simulink model "Single_Phase_PWM_Dual_Inverter_grid_R2023a"  (R2023a)
settings: Solver=ode45  StartTime=0.0  StopTime=0.2  RelTol=1e-3
libraries: spsMosfetLib x8, spsSeriesRLCBranchLib x7, spsCurrentMeasurementLib x3, spsDCVoltageSourceLib x2, spsPLLLib x2, spsPWMGenerator2LevelLib x2, spsVoltageMeasurementLib x2, spsACVoltageSourceLib x1, spspowerguiLib x1
settings Model: Creator=JD  LastModifiedBy=JD
settings DebuggingCC: UnconnectedInputMsg=warning  UnconnectedOutputMsg=warning  UnconnectedLineMsg=warning
settings ModelReferenceCC: EnableRefExpFcnMdlSchedulingChecks=on
settings RTWCC: DLArmComputeVersion=19.05

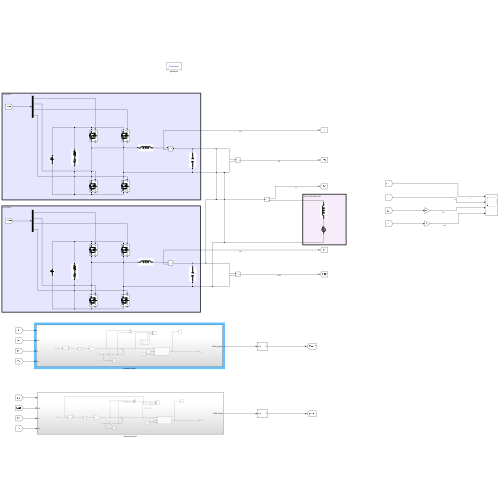
[thumbnail: Simulink's stored preview of the top-level diagram]
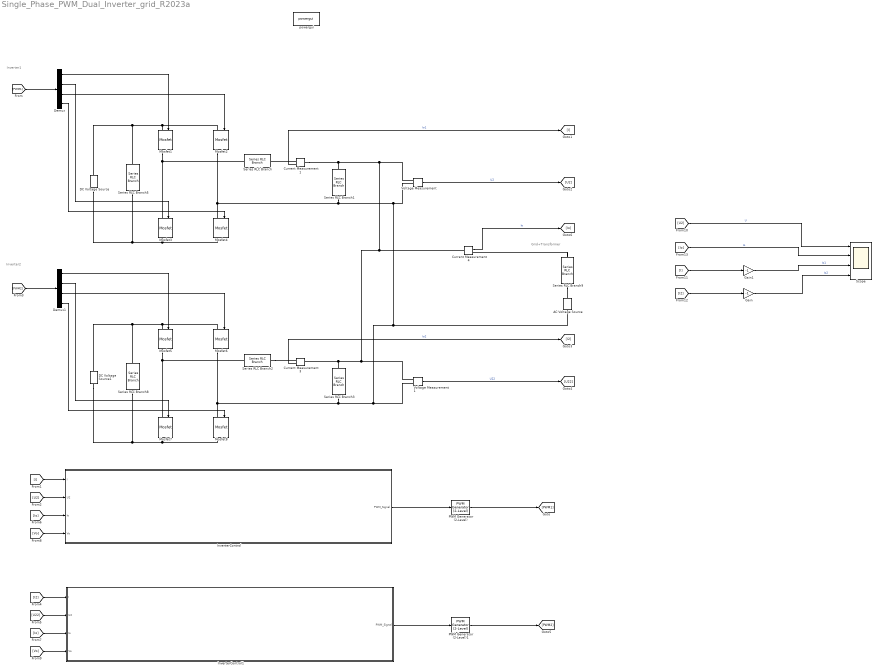
== system Single_Phase_PWM_Dual_Inverter_grid_R2023a ==
  note: Grid+Transformer
  note: Inverter2
  note: Inverter1
  AC Voltage Source : spsACVoltageSourceLib/AC Voltage Source  Amplitude=24*sqrt(2)  Phase=0  Frequency=50  SampleTime=0  Measurements=None  BusType=swing  Pref=10e3  Qref=0  Qmin=-inf  Qmax=+inf
  Current Measurement1 : spsCurrentMeasurementLib/Current Measurement  PhasorSimulation=off  OutputType=Complex  PSBequivalent=0
  Current Measurement3 : spsCurrentMeasurementLib/Current Measurement  PhasorSimulation=off  OutputType=Complex  PSBequivalent=0
  Current Measurement4 : spsCurrentMeasurementLib/Current Measurement  PhasorSimulation=off  OutputType=Complex  PSBequivalent=0
  DC Voltage Source : spsDCVoltageSourceLib/DC Voltage Source  Amplitude=48  Measurements=None
  DC Voltage Source1 : spsDCVoltageSourceLib/DC Voltage Source  Amplitude=48  Measurements=None
  Demux : Demux
  Demux1 : Demux
  Gain : Gain  Gain=-1
  Gain1 : Gain  Gain=-1
  InverterControl : Subsystem
  InverterControl1 : Subsystem
  Mosfet{1..8} (8 alike) : spsMosfetLib/Mosfet  Ron=0.1  Lon=0  Rd=0.01  Vfd=0  IC=0  Rs=1e5  Cs=inf  Measurements=on
  PWM Generator (2-Level) : spsPWMGenerator2LevelLib/PWM Generator (2-Level)  ModulatorType=Single-phase full-bridge (4 pulses)  ModulatorMode=Unsynchronized  Fc=20000  Pc=90  nF=27  MinMax="[ -1  1 ]"  SamplingTechnique=Natural  ModulatingSignals=off  m=0.8  Freq=60  Phase=0  Ts=0  ShowCarrierOutport=off
  PWM Generator (2-Level)1 : spsPWMGenerator2LevelLib/PWM Generator (2-Level)  ModulatorType=Single-phase full-bridge (4 pulses)  ModulatorMode=Unsynchronized  Fc=20000  Pc=90  nF=27  MinMax="[ -1  1 ]"  SamplingTechnique=Natural  ModulatingSignals=off  m=0.8  Freq=60  Phase=0  Ts=0  ShowCarrierOutport=off
  Scope : Scope  NumInputPorts=4
  Series RLC Branch : spsSeriesRLCBranchLib/Series RLC Branch  LConnTagsString=__new0  RConnTagsString=__new0  BranchType=L  Resistance=1  Inductance=1e-3  SetiL0=off  InitialCurrent=0  Capacitance=1e-6  Setx0=off  InitialVoltage=0  Measurements=None
  Series RLC Branch1 : spsSeriesRLCBranchLib/Series RLC Branch  LConnTagsString=__new0  RConnTagsString=__new0  BranchType=C  Resistance=1  Inductance=1e-3  SetiL0=off  InitialCurrent=0  Capacitance=4.7e-6  Setx0=off  InitialVoltage=0  Measurements=None
  Series RLC Branch2 : spsSeriesRLCBranchLib/Series RLC Branch  LConnTagsString=__new0  RConnTagsString=__new0  BranchType=L  Resistance=1  Inductance=1e-3  SetiL0=off  InitialCurrent=0  Capacitance=1e-6  Setx0=off  InitialVoltage=0  Measurements=None
  Series RLC Branch3 : spsSeriesRLCBranchLib/Series RLC Branch  LConnTagsString=__new0  RConnTagsString=__new0  BranchType=C  Resistance=1  Inductance=1e-3  SetiL0=off  InitialCurrent=0  Capacitance=4.7e-6  Setx0=off  InitialVoltage=0  Measurements=None
  Series RLC Branch5 : spsSeriesRLCBranchLib/Series RLC Branch  LConnTagsString=__new0  RConnTagsString=__new0  BranchType=RC  Resistance=0.0001  Inductance=1e-3  SetiL0=off  InitialCurrent=0  Capacitance=940e-6  Setx0=off  InitialVoltage=0  Measurements=None
  Series RLC Branch8 : spsSeriesRLCBranchLib/Series RLC Branch  LConnTagsString=__new0  RConnTagsString=__new0  BranchType=RC  Resistance=0.0001  Inductance=1e-3  SetiL0=off  InitialCurrent=0  Capacitance=940e-6  Setx0=off  InitialVoltage=0  Measurements=None
  Series RLC Branch9 : spsSeriesRLCBranchLib/Series RLC Branch  LConnTagsString=__new0  RConnTagsString=__new0  BranchType=L  Resistance=1  Inductance=100e-6  SetiL0=off  InitialCurrent=0  Capacitance=1e-6  Setx0=off  InitialVoltage=0  Measurements=None
  Voltage Measurement : spsVoltageMeasurementLib/Voltage Measurement  PhasorSimulation=off  OutputType=Complex  PSBequivalent=0
  Voltage Measurement1 : spsVoltageMeasurementLib/Voltage Measurement  PhasorSimulation=off  OutputType=Complex  PSBequivalent=0
  powergui : spspowerguiLib/powergui  Priority=1  SimulationMode=Continuous  SampleTime=1e-6  frequency=60  Iterations=50  frequencyindice=0  Pbase=100e6  ErrMax=1e-4  UnitsV=kV  UnitsW=MW  buscounter=0  FunctionMessages=off  echomessages=off  EnableUseOfTLC=off  CurrentSourceSwitches=off  DisableSnubberDevices=off  DisableRonSwitches=off  DisableVfSwitches=off  DisplayEquations=off  AutomaticDiscreteSolvers=off  SolverType=Tustin/Backward Euler (TBE)  Interpol=off  ExternalGateDelay=off  methode=off  Ts=100  x0status=blocks  SPID=on  SwTol=0  HookPort=off  NonlinearTolerance=1e-4  nMaxIteration=100  ContinueOnMaxIteration=off  RestoreLinks=warning  ResistiveCurrentMeasurement=off  Frange=[0:2:500]  Ylog=off  Xlog=on  ShowGrid=off  save=off  variable=ZData  structure=0  ZoomFFT=off  StartTime=0.0  cycles=1  DisplayStyle=1  fundamental=60  FreqAxis=off  MaxFrequency=1000  frequencyindicesteady=1  RmsSteady=1  display=off
  wires:
  Voltage Measurement/1 -> [U2]  "U2"
  [PWM1] -> Demux/1
  Demux/1 -> Mosfet1/1
  Demux/2 -> Mosfet3/1
  Demux/3 -> Mosfet2/1
  Demux/4 -> Mosfet4/1
  PWM Generator (2-Level)/1 -> [PWM1]
  Current Measurement1/1 -> [I]  "Io1"
  [I] -> InverterControl/1(I)
  [U2] -> InverterControl/2(U2)
  InverterControl/1(PWM_Signal) -> PWM Generator (2-Level)/1
  Current Measurement3/1 -> [I2]  "Io2"
  Demux1/4 -> Mosfet8/1
  Demux1/3 -> Mosfet6/1
  Demux1/2 -> Mosfet7/1
  Demux1/1 -> Mosfet5/1
  [PWM2] -> Demux1/1
  Voltage Measurement1/1 -> [U22]  "U22"
  InverterControl1/1(PWM_Signal) -> PWM Generator (2-Level)1/1
  [U22] -> InverterControl1/2(U2)
  [I2] -> InverterControl1/1(I)
  Current Measurement4/1 -> [Io]  "Io"
  [Io] -> InverterControl/3(Io)
  [Io] -> InverterControl1/3(Io)
  [Vo] -> InverterControl/4(Vo)
  [Vo] -> InverterControl1/4(Vo)
  PWM Generator (2-Level)1/1 -> [PWM2]
  [U2] -> Scope/1  "U"
  [I] -> Gain1/1
  [I2] -> Gain/1
  [Io] -> Scope/2  "Io"
  Gain1/1 -> Scope/3  "Io1"
  Gain/1 -> Scope/4  "Io2"
  connections:
  Mosfet2/LConn1 -- DC Voltage Source/RConn1 -- Series RLC Branch5/LConn1 -- Mosfet1/LConn1
  Mosfet4/RConn1 -- DC Voltage Source/LConn1 -- Series RLC Branch5/RConn1 -- Mosfet3/RConn1
  Mosfet1/RConn1 -- Mosfet3/LConn1 -- Series RLC Branch/LConn1
  Current Measurement1/RConn1 -- Series RLC Branch/RConn1
  Mosfet6/RConn1 -- Mosfet8/LConn1 -- Series RLC Branch3/RConn1 -- AC Voltage Source/LConn1 -- Mosfet2/RConn1 -- Mosfet4/LConn1 -- Series RLC Branch1/RConn1 -- Voltage Measurement/LConn2 -- Voltage Measurement1/LConn2
  Series RLC Branch9/LConn1 -- Current Measurement4/RConn1
  Mosfet6/LConn1 -- DC Voltage Source1/RConn1 -- Series RLC Branch8/LConn1 -- Mosfet5/LConn1
  Mosfet8/RConn1 -- Series RLC Branch8/RConn1 -- DC Voltage Source1/LConn1 -- Mosfet7/RConn1
  Mosfet5/RConn1 -- Series RLC Branch2/LConn1 -- Mosfet7/LConn1
  Series RLC Branch2/RConn1 -- Current Measurement3/RConn1
  Voltage Measurement1/LConn1 -- Current Measurement4/LConn1 -- Current Measurement1/LConn1 -- Series RLC Branch1/LConn1 -- Voltage Measurement/LConn1 -- Current Measurement3/LConn1 -- Series RLC Branch3/LConn1
  Series RLC Branch9/RConn1 -- AC Voltage Source/RConn1

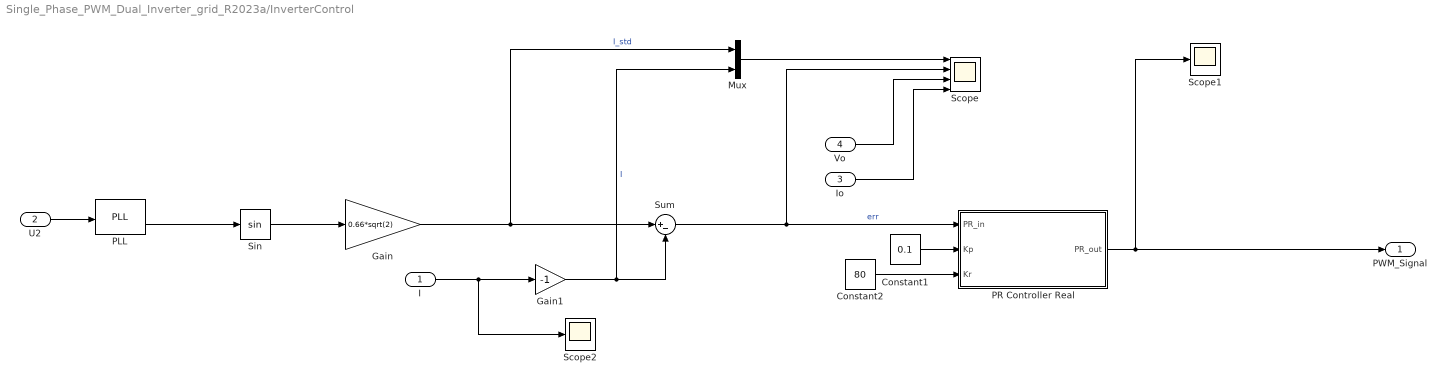
== system Single_Phase_PWM_Dual_Inverter_grid_R2023a/InverterControl ==
  I : Inport
  U2 : Inport  Port=2
  Io : Inport  Port=3
  Vo : Inport  Port=4
  Constant1 : Constant  Value=0.1
  Constant2 : Constant  Value=80
  Gain : Gain  Gain=0.66*sqrt(2)
  Gain1 : Gain  Gain=-1
  Mux : Mux  Inputs=2
  PLL : spsPLLLib/PLL  Fmin=45  Par_Init=[0, 50]  ParK=[180, 3200, 1]  TcD=1e-4  MaxRateChangeFreq=12  FilterCutOffFreq=25  Ts=0  AGC=on
  PR Controller Real : Subsystem
  Scope : Scope  NumInputPorts=4
  Scope1 : Scope
  Scope2 : Scope
  Sin : Trigonometry
  Sum : Sum  Inputs=|+-
  PWM_Signal : Outport
  wires:
  Constant1/1 -> PR Controller Real/2(Kp)
  Constant2/1 -> PR Controller Real/3(Kr)
  Mux/1 -> Scope/1
  Sum/1 -> PR Controller Real/1(PR_in), Scope/2  "err"
  PR Controller Real/1(PR_out) -> PWM_Signal/1, Scope1/1
  I/1 -> Scope2/1, Gain1/1
  Io/1 -> Scope/4
  Gain1/1 -> Sum/2, Mux/2  "I"
  U2/1 -> PLL/1
  PLL/2 -> Sin/1
  Sin/1 -> Gain/1
  Gain/1 -> Mux/1, Sum/1  "I_std"
  Vo/1 -> Scope/3

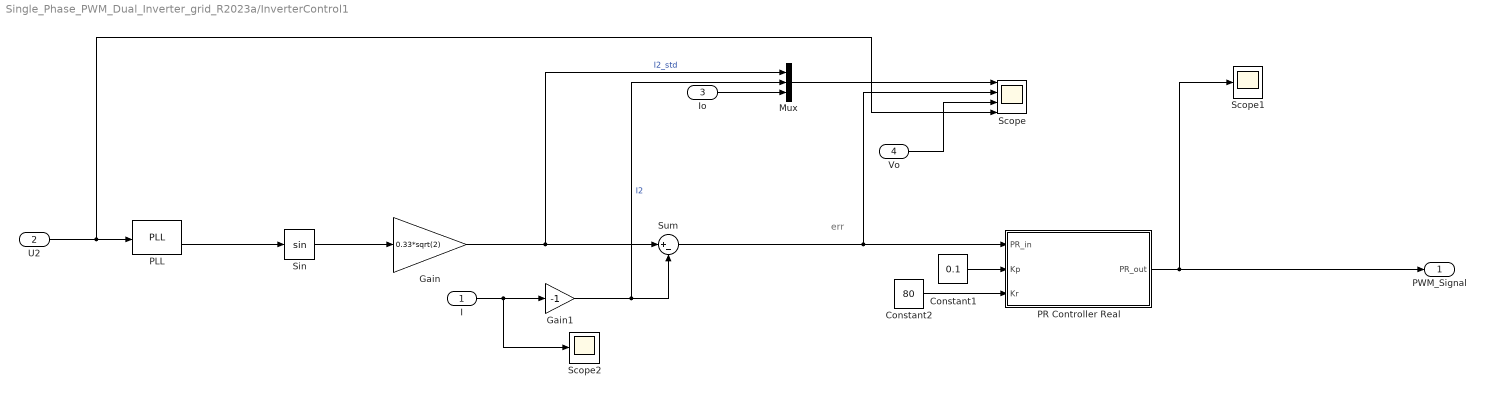
== system Single_Phase_PWM_Dual_Inverter_grid_R2023a/InverterControl1 ==
  note: err
  I : Inport
  U2 : Inport  Port=2
  Io : Inport  Port=3
  Vo : Inport  Port=4
  Constant1 : Constant  Value=0.1
  Constant2 : Constant  Value=80
  Gain : Gain  Gain=0.33*sqrt(2)
  Gain1 : Gain  Gain=-1
  Mux : Mux  Inputs=3
  PLL : spsPLLLib/PLL  Fmin=45  Par_Init=[0, 50]  ParK=[180, 3200, 1]  TcD=1e-4  MaxRateChangeFreq=12  FilterCutOffFreq=25  Ts=0  AGC=on
  PR Controller Real : Subsystem
  Scope : Scope  NumInputPorts=4
  Scope1 : Scope
  Scope2 : Scope
  Sin : Trigonometry
  Sum : Sum  Inputs=|+-
  PWM_Signal : Outport
  wires:
  U2/1 -> Scope/4, PLL/1
  I/1 -> Scope2/1, Gain1/1
  PR Controller Real/1(PR_out) -> Scope1/1, PWM_Signal/1
  Sum/1 -> Scope/2, PR Controller Real/1(PR_in)
  Mux/1 -> Scope/1
  Constant2/1 -> PR Controller Real/3(Kr)
  Constant1/1 -> PR Controller Real/2(Kp)
  PLL/2 -> Sin/1
  Vo/1 -> Scope/3
  Gain/1 -> Mux/1, Sum/1  "I2_std"
  Sin/1 -> Gain/1
  Gain1/1 -> Sum/2, Mux/2  "I2"
  Io/1 -> Mux/3

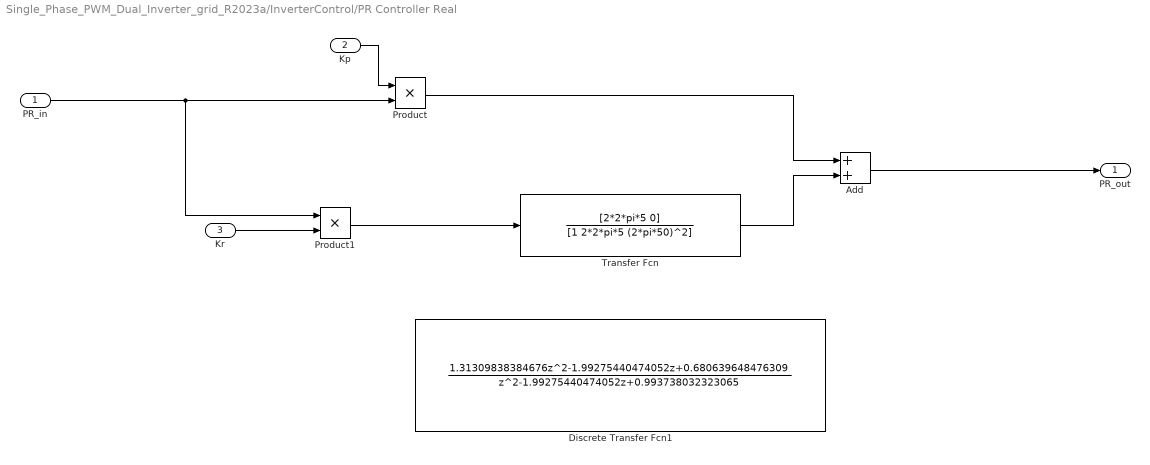
== system Single_Phase_PWM_Dual_Inverter_grid_R2023a/InverterControl/PR Controller Real ==
  PR_in : Inport
  Kp : Inport  Port=2
  Kr : Inport  Port=3
  Add : Sum
  Discrete Transfer Fcn1 : DiscreteTransferFcn  Numerator=[1.31309838384676 -1.99275440474052 0.680639648476309]  Denominator=[1 -1.99275440474052 0.993738032323065]  SampleTime=0.0001
  Product : Product
  Product1 : Product
  Transfer Fcn : TransferFcn  Numerator=[2*2*pi*5 0]  Denominator=[1 2*2*pi*5 (2*pi*50)^2]
  PR_out : Outport
  wires:
  Transfer Fcn/1 -> Add/2
  Kp/1 -> Product/1
  Product1/1 -> Transfer Fcn/1
  Kr/1 -> Product1/2
  Product/1 -> Add/1
  PR_in/1 -> Product/2, Product1/1
  Add/1 -> PR_out/1

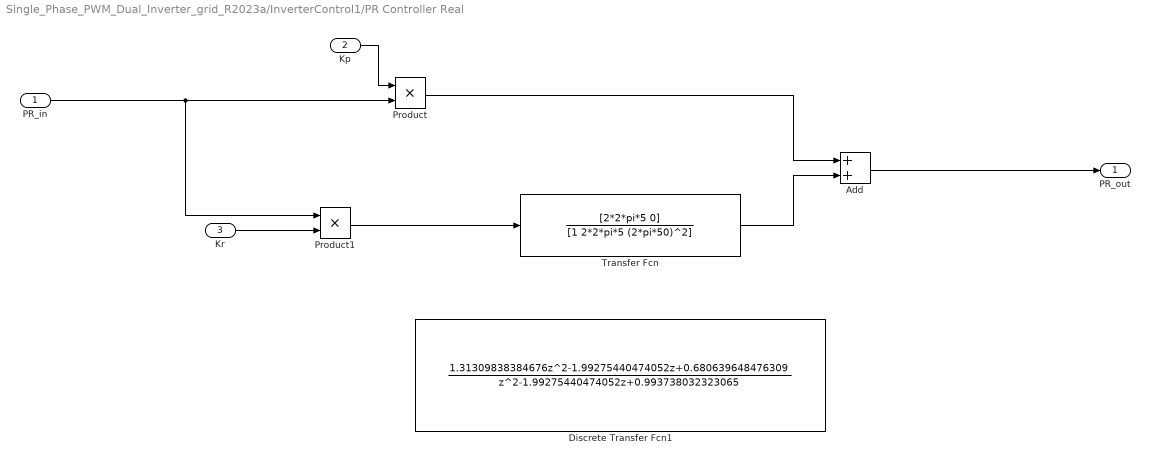
== system Single_Phase_PWM_Dual_Inverter_grid_R2023a/InverterControl1/PR Controller Real ==
  PR_in : Inport
  Kp : Inport  Port=2
  Kr : Inport  Port=3
  Add : Sum
  Discrete Transfer Fcn1 : DiscreteTransferFcn  Numerator=[1.31309838384676 -1.99275440474052 0.680639648476309]  Denominator=[1 -1.99275440474052 0.993738032323065]  SampleTime=0.0001
  Product : Product
  Product1 : Product
  Transfer Fcn : TransferFcn  Numerator=[2*2*pi*5 0]  Denominator=[1 2*2*pi*5 (2*pi*50)^2]
  PR_out : Outport
  wires:
  Add/1 -> PR_out/1
  PR_in/1 -> Product1/1, Product/2
  Product/1 -> Add/1
  Kr/1 -> Product1/2
  Product1/1 -> Transfer Fcn/1
  Kp/1 -> Product/1
  Transfer Fcn/1 -> Add/2
